simulink model "ss51"  (R2013a)
settings: Solver=ode45  StartTime=0.0  StopTime=50  FixedStep=T  RelTol=1e-3
values from neighbouring files (symbols this model uses):
  A = [0 1; 0 0]    [ss1_init.m]    (also in ss512_init.m = [0 0 1 0; ss51_init.m = [0 0 1 0)
  B = [0; 1]    [ss1_init.m]    (also in ss512_init.m = [0; 0; 0; 1]; ss51_init.m = [0; 0; 0; 1])
  C = eye(2)    [ss1_init.m]    (also in ss512_init.m = eye(n); ss51_init.m = eye(n))
  D = [0; 0]    [ss1_init.m]    (also in ss512_init.m = zeros([n 1]); ss51_init.m = zeros([n 1]))
  K1 = myacker(Phi, Gamma, z1)    [ss512_init.m]    (also in ss51_init.m)
  K2 = myacker(Phi, Gamma, z2)    [ss512_init.m]    (also in ss51_init.m)
  T = 0.1    [ex8_init.m]    (also in ss1_init.m; ss512_init.m = 0.4; ss51_init.m = 0.4)
  x1 = [1; 0]    [ex8_init.m]    (also in ss1_init.m = [1; 1]; ss512_init.m = [1; 0; 0; 0]; ss51_init.m = [1; 0; 0; 0])
settings Model: Creator=jmahler  LastModifiedBy=jmahler

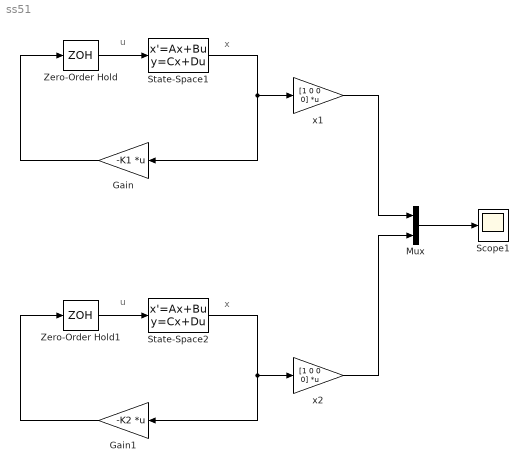
== system ss51 ==
  note: u
  note: x
  note: u
  note: x
  Gain : Gain  Gain=-K1  Multiplication=Matrix(K*u)
  Gain1 : Gain  Gain=-K2  Multiplication=Matrix(K*u)
  Mux : Mux  Inputs=2
  Scope1 : Scope
  State-Space1 : StateSpace  A=A  B=B  C=C  D=D  X0=x1
  State-Space2 : StateSpace  A=A  B=B  C=C  D=D  X0=x1
  Zero-Order Hold : ZeroOrderHold  SampleTime=T
  Zero-Order Hold1 : ZeroOrderHold  SampleTime=T
  x1 : Gain  Gain=[1 0 0 0]  Multiplication=Matrix(K*u)
  x2 : Gain  Gain=[1 0 0 0]  Multiplication=Matrix(K*u)
  wires:
  Gain/1 -> Zero-Order Hold/1
  Zero-Order Hold/1 -> State-Space1/1
  State-Space1/1 -> x1/1, Gain/1
  Gain1/1 -> Zero-Order Hold1/1
  Zero-Order Hold1/1 -> State-Space2/1
  State-Space2/1 -> x2/1, Gain1/1
  Mux/1 -> Scope1/1
  x1/1 -> Mux/1
  x2/1 -> Mux/2
